simulink model "E55_1030"  (R2019b)
settings: Solver=FixedStepDiscrete  StartTime=0.0  StopTime=10  FixedStep=0.0005  RelTol=1e-3  EnableMultiTasking=on
InitFcn:
  | ecucoder_canfd
  | load('DATA_Plimit.mat')
  | a=0.775;
  | b=0.775;
  | kf=-50000;
  | kr=-50000;
  | m=226+75;
  | Iz=100;
  | u=0.85;
  | g=9.8;
  | L=a+b;
  | xi=0.1;
  | r=0.226;
  | Lw=1.171;
  | Tm=21;
  | i=15.9;
  | Jw=0.504;
  | Pmax=20000;
  | mw=19.3;
  | mb=148.9+75;
  | hg=0.280;
model workspace (MAT data in the model file):
  Initial_Steer_Position = 0
values from neighbouring files (symbols this model uses):
  SOC = [2.5 5 7.5 10 20 30 40 50 60 70 80 90 ... (14 elements, 14x1)]    [DATA_Plimit.mat]
  SOC_Discharge = [2.04592350211 2.57821618825 3.10671863859 3.63118835861 4.15200192786 4.66837694959 5.18149950051 5.69046162564 6.19532286188 6.696400261 7.19347596839 7.68712157998 ... (473 elements, 1x473)]    [DATA_Plimit.mat]
  VOLTAGE = [459.1488 476.0844 485.9448 487.344 492.822 498.8016 503.382 509.1108 518.8128 531.2472 544.5132 558.4656 ... (14 elements, 14x1)]    [DATA_Plimit.mat]
undefined symbols (not defined in the file or in its folder): DiscIntNeverNeededParam, H, HALL10, HALL6, HALL7, HALL8, HALL9, HPWM1, HPWM3, I_AN05_5V, I_AN07_5V, I_AN08_5V, I_AN09_5V, I_AN10_5V, I_SW11_H, I_SW12_H, I_SW13_H, I_SW14_H, I_SW15_H, I_SW16_H, I_SW17_H, I_SW18_H, I_SW19_H, LS1A2, O_HS1A2, O_HS1A8
libraries: ec311lib x152, simulink x92, canmsglib x30, canfdmsglib x2
(part 2 of 6)

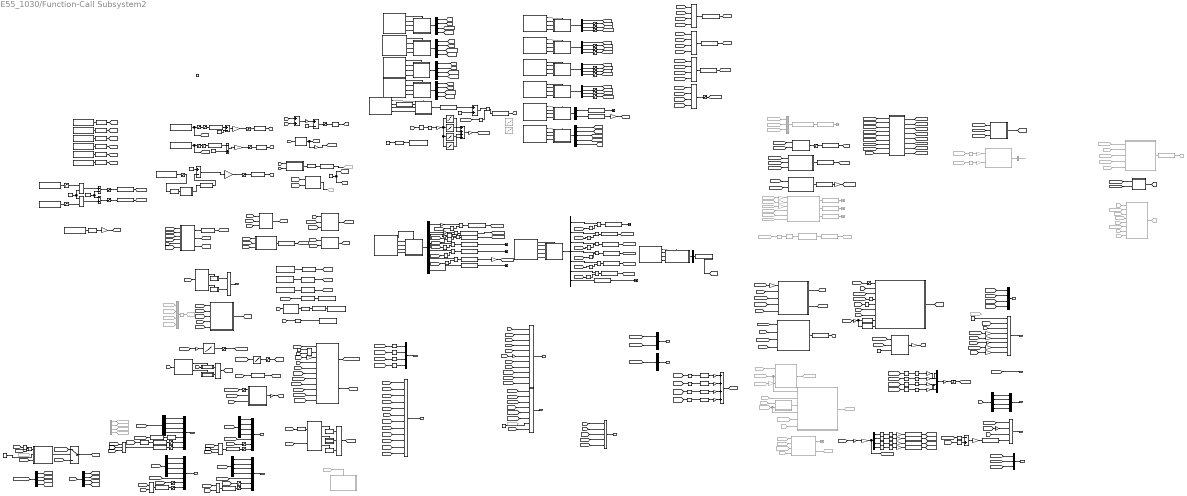
== system E55_1030/Function-Call Subsystem2 ==
  note: 三个地方要改
  note: 坐标变换（计算不带重力加速度的加速度）
  note: K3105G数据前置处理
  note: 数据滤波
  note: 此算法中量的单位：速度（m/s）、角度角速度（rad、rad/s）、轮速（rpm）
  note: 扭矩分配和驱动防滑
  note: 状态机
  note: 传感器数据接收
  note: 低压电池电压检测
  note: Yaw_Rate、Side_Slip_Angle、Steer_Angle都以向左转为正（逆时针）
  note: 设置速度
      | 待驶：0 前进：20000 倒车：-5000
  note: BMS CAN发送
  note: 功率限制
  note: 信息传输给仪表盘
  note: 精度不如IMU测的角速度
  note: 刹车油压传感器
  note: 安全回路状态检测
  note: IO输入输出
  note: 几个角度的定义，Heading和Yaw以顺时针为正，Side Slip以逆时针为正
      | Yaw Angle和Heading Angle取值为0到360°，Side Slip Angle取值为-180到180°
  note: 油门输入及可靠检测
  note: 新版CAN发送
      | 参数传入AMK
  note: 开环扭矩分配和动能回收
  note: 屏幕控制信息_55E
      | (控制K3105是否打开)
  note: 发1关闭K3105
  note: CAN接收
  note: 旋转顺序： yaw-pitch-roll
  note: XYZ：右前上
      | Yaw绕Z（左手系），Roll绕Y（右手系），Pitch绕X（右手系）
      | 加速度：XYZ正方向为负
      | Yaw：Y轴正方向和正北方向的夹角
      | Yaw_Rate：车头向左为正（右手系）
  function : TriggerPort  TriggerType=function-call  VariantControl=Variant
  1-D Lookup Table : Lookup_n-D  Commented=on  NumberOfTableDimensions=1  BreakpointsForDimension1=[-100,-60,-30.4,0,30,60,95]  Table=[-14.489,-10.473,-5.315,0,6.137,12.407,14.976]  InternalRulePriority=Speed  RndMeth=Simplest  InputSameDT=on
  1-D Lookup Table1 : Lookup_n-D  NumberOfTableDimensions=1  BreakpointsForDimension1=[0,100]  Table=[25000,36000]  InternalRulePriority=Speed  RndMeth=Simplest  InputSameDT=on
  1-D Lookup Table2 : Lookup_n-D  Commented=on  NumberOfTableDimensions=1  BreakpointsForDimension1=[-98.8,-60,-30,0,30,60,91.7]  Table=[-15.376,-12.134,-8.11,0,4.475,10.343,13.631]  InternalRulePriority=Speed  RndMeth=Simplest  InputSameDT=on
  AMKSpeed10 : canmsglib/CAN Pack  Commented=on  MsgList=(none)  MsgName=ESC_5_RearWhlSpdKPH  MsgIDType=Standard (11-bit identifier)  MsgIdentifier=291  MsgLength=8  Remote=off  ApplyMinMax=off  BusOutput=on  SignalInfo={ 'ESC_WheelSpeedKph_RL', '8', '13', 'BE', 'unsigned', 'Standard', '0', '0.05625', '0', '0', '460.6875'; 'ESC_WheelSpeedKph_RR', '24', '13', 'BE', 'unsigned', 'Standard', '0', '0.05625', '0', '0', '460.6875' }
      settings: SourceProductName=Vehicle Network Toolbox  SourceProductBaseCode=VN  DataFormat=manually specified signals
  AMK复位开关 : ec311lib/RapidECU_U34/01BasicInput/SwitchInput  channel=103:I_SW19_H/HALL10  sampletime=-1
      settings: SourceProductName=ECUCoder for S32K311
  Abs{,1..7} (8 alike) : Abs
  Abs10 : Abs  Commented=on
  Abs8 : Abs  Commented=on
  Abs9 : Abs  Commented=on
  Add : Sum  Inputs=++++
  Add1 : Sum
  Add2 : Sum  Inputs=+-
  Add3 : Sum  Inputs=+-
  Add4 : Sum  Inputs=-+
  Add5 : Sum
  AnalogInput : ec311lib/RapidECU_U34/01BasicInput/AnalogInput  channel=55:I_AN08_5V  sampletime=-1
      settings: SourceProductName=ECUCoder for S32K311
  AnalogInput1 : ec311lib/RapidECU_U34/01BasicInput/AnalogInput  channel=56:I_AN09_5V  sampletime=-1
      settings: SourceProductName=ECUCoder for S32K311
  BRAKE_HIGH1 : Constant  Value=1153
  Bus Creator{,6..7,14} (4 alike) : BusCreator  Inputs=4
  Bus Creator{1..4} (4 alike) : BusCreator  Inputs=7
  Bus Creator10 : BusCreator  Inputs=8
  Bus Creator11 : BusCreator  Inputs=1
  Bus Creator12 : BusCreator  Inputs=2
  Bus Creator13 : BusCreator  Inputs=3
  Bus Creator15 : BusCreator  Inputs=5
  Bus Creator5 : BusCreator  Inputs=8
  Bus Creator8 : BusCreator  Inputs=12
  Bus Creator9 : BusCreator  Inputs=11
  Bus Selector : BusSelector  OutputSignals=K3105_Alive
  Bus Selector1 : BusSelector  OutputSignals=INS_IMUAccrnX,INS_IMUAccrnY,INS_IMUAccrnZ,INS_IMUAglRateX,INS_IMUAglRateY,INS_IMUAglRateZ,CAN_OK
  Bus Selector{8..11} (4 alike) : BusSelector  OutputSignals=ErrorCode,TempIGBT,TempInverter,TempMotor
  Bus Selector12 : BusSelector  OutputSignals=IVT_MsgCount,IVT_Msg_Result_W
  Bus Selector13 : BusSelector  OutputSignals=BMSState,CellTemp,MaxCellVolt,MinCellVolt,SOC
  Bus Selector{18,20,22,24} (4 alike) : BusSelector  OutputSignals=DcOn,Enable,ErrorReset,InverterOn
  Bus Selector2 : BusSelector  OutputSignals=To_Ground_Speed,East_Speed,North_Speed,Heading_Angle,Pitch_Angle,Roll_Angle,CAN_OK
  Bus Selector27 : BusSelector  Commented=on  OutputSignals=Data
  Bus Selector{3..6} (4 alike) : BusSelector  OutputSignals=Id,Iq,AMK_Speed,bError
  CAN0to2Receive : ec311lib/RapidECU_U34/03CANCommunication/CAN0to2Receive  canmodule=2  canbuffer=56  canmessageid=hex2dec('0283')  canmessagetype=Standard(11-bit ID)  datalength=8  sampletime=-1
      settings: SourceProductName=ECUCoder for S32K311
  CAN0to2Receive1 : ec311lib/RapidECU_U34/03CANCommunication/CAN0to2Receive  canmodule=2  canbuffer=57  canmessageid=hex2dec('0284')  canmessagetype=Standard(11-bit ID)  datalength=8  sampletime=-1
      settings: SourceProductName=ECUCoder for S32K311
  CAN0to2Receive10 : ec311lib/RapidECU_U34/03CANCommunication/CAN0to2Receive  canmodule=0  canbuffer=20  canmessageid=hex2dec('055A')  canmessagetype=Standard(11-bit ID)  datalength=8  sampletime=-1
      settings: SourceProductName=ECUCoder for S32K311
  CAN0to2Receive13 : ec311lib/RapidECU_U34/03CANCommunication/CAN0to2Receive  canmodule=0  canbuffer=21  canmessageid=hex2dec('055E')  canmessagetype=Standard(11-bit ID)  datalength=8  sampletime=-1
      settings: SourceProductName=ECUCoder for S32K311
  CAN0to2Receive2 : ec311lib/RapidECU_U34/03CANCommunication/CAN0to2Receive  canmodule=2  canbuffer=58  canmessageid=hex2dec('0287')  canmessagetype=Standard(11-bit ID)  datalength=8  sampletime=-1
      settings: SourceProductName=ECUCoder for S32K311
  CAN0to2Receive3 : ec311lib/RapidECU_U34/03CANCommunication/CAN0to2Receive  canmodule=2  canbuffer=59  canmessageid=hex2dec('0288')  canmessagetype=Standard(11-bit ID)  datalength=8  sampletime=-1
      settings: SourceProductName=ECUCoder for S32K311
  CAN0to2Receive4 : ec311lib/RapidECU_U34/03CANCommunication/CAN0to2Receive  canmodule=2  canbuffer=60  canmessageid=hex2dec('0285')  canmessagetype=Standard(11-bit ID)  datalength=8  sampletime=-1
      settings: SourceProductName=ECUCoder for S32K311
  CAN0to2Receive5 : ec311lib/RapidECU_U34/03CANCommunication/CAN0to2Receive  canmodule=2  canbuffer=61  canmessageid=hex2dec('0286')  canmessagetype=Standard(11-bit ID)  datalength=8  sampletime=-1
      settings: SourceProductName=ECUCoder for S32K311
  CAN0to2Receive6 : ec311lib/RapidECU_U34/03CANCommunication/CAN0to2Receive  canmodule=2  canbuffer=62  canmessageid=hex2dec('0289')  canmessagetype=Standard(11-bit ID)  datalength=8  sampletime=-1
      settings: SourceProductName=ECUCoder for S32K311
  CAN0to2Receive7 : ec311lib/RapidECU_U34/03CANCommunication/CAN0to2Receive  canmodule=2  canbuffer=63  canmessageid=hex2dec('028A')  canmessagetype=Standard(11-bit ID)  datalength=8  sampletime=-1
      settings: SourceProductName=ECUCoder for S32K311
  CAN0to2Receive8 : ec311lib/RapidECU_U34/03CANCommunication/CAN0to2Receive  canmodule=0  canbuffer=35  canmessageid=hex2dec('01E5')  canmessagetype=Standard(11-bit ID)  datalength=8  sampletime=-1
      settings: SourceProductName=ECUCoder for S32K311
  CAN0to2Receive9 : ec311lib/RapidECU_U34/03CANCommunication/CAN0to2Receive  canmodule=0  canbuffer=24  canmessageid=hex2dec('0526')  canmessagetype=Standard(11-bit ID)  datalength=6  sampletime=-1
      settings: SourceProductName=ECUCoder for S32K311
  CAN5WakeUp : ec311lib/RapidECU_U34/03CANCommunication/CAN5WakeUp  channel=CAN5WakeUp  sampletime=-1
      settings: SourceProductName=ECUCoder for S32K311
  Constant{,5..7} (4 alike) : Constant
  Constant10 : Constant  Value=0
  Constant11 : Constant  Value=0
  Constant2 : Constant  Value=-377
  Constant25 : Constant  Value=3.125
  Constant3 : Constant  Value=3271
  Constant36 : Constant  Value=160
  Constant4 : Constant  Value=5
  Constant8 : Constant  Value=0
  Constant9 : Constant  Value=1433
  Data Type Conversion{,1,5,7..9,12..13} (8 alike) : DataTypeConversion
  Data Type Conversion10 : DataTypeConversion  OutDataTypeStr=boolean
  Data Type Conversion11 : DataTypeConversion  OutDataTypeStr=int16  RndMeth=Nearest
  Data Type Conversion14 : DataTypeConversion  OutDataTypeStr=boolean
  Data Type Conversion2 : DataTypeConversion  RndMeth=Nearest
  Data Type Conversion6 : DataTypeConversion  OutDataTypeStr=boolean
  Demux{,1,3..4} (4 alike) : Demux
  Demux2 : Demux  Commented=on
  Difference : simulink/Discrete/Difference  Commented=on  ICPrevInput=0.0  OutMin=[]  OutMax=[]  OutDataType=fixdt(1, 16)  OutScaling=2^-10  DoSatur=off
  Divide5 : Product  Inputs=/*
  Divide7 : Product  Inputs=*/
  Fcn1 : Fcn  Commented=on  Expr=sqrt(u(1)*u(1)+u(2)*u(2)+u(3)*u(3))
  From15 : From  Commented=on  GotoTag=reset_input
  From158 : From  Commented=on  GotoTag=Wheel_Steer_Angle
  From170 : From  Commented=on  GotoTag=Yaw_Rate_d
  From171 : From  Commented=on  GotoTag=wheel_speed_d
  From172 : From  Commented=on  GotoTag=wheel_speed_d
  From174 : From  Commented=on  GotoTag=wheel_speed
  From177 : From  Commented=on  GotoTag=velocity
  From182 : From  Commented=on  GotoTag=wheel_speed
  From183 : From  Commented=on  GotoTag=Torque_Dis
  From184 : From  Commented=on  GotoTag=Torque_ASR
  From197 : From  Commented=on  GotoTag=T_max_d
  From207 : From  Commented=on  GotoTag=INS_IMUAccrnY_filter
  From221 : From  Commented=on  GotoTag=Algorithm_Enable
  From224 : From  Commented=on  GotoTag=Algorithm_Enable
  From232 : From  Commented=on  GotoTag=AMKSpeed_RR
  From233 : From  Commented=on  GotoTag=AMKSpeed_FL
  From234 : From  Commented=on  GotoTag=AMKSpeed_FR
  From235 : From  Commented=on  GotoTag=AMKSpeed_RL
  From239 : From  Commented=on  GotoTag=Yaw_Rate_d
  From240 : From  Commented=on  GotoTag=Yaw_Rate_d
  From241 : From  Commented=on  GotoTag=Wheel_Steer_Angle
  From242 : From  Commented=on  GotoTag=velocity
  From243 : From  Commented=on  GotoTag=Side_Slip_Angle
  From244 : From  Commented=on  GotoTag=Yaw_Rate_filter
  From245 : From  Commented=on  GotoTag=Fz
  From246 : From  Commented=on  GotoTag=break
  From247 : From  Commented=on  GotoTag=Wheel_Steer_Angle
  From248 : From  Commented=on  GotoTag=Torque_req
  From25 : From  Commented=on  GotoTag=INS_IMUAccrnX
  From252 : From  Commented=on  GotoTag=T_max_d
  From255 : From  Commented=on  GotoTag=Mz_r
  From26 : From  Commented=on  GotoTag=Yaw_Rate_filter
  From27 : From  Commented=on  GotoTag=INS_IMUAccrnY
  From28 : From  Commented=on  GotoTag=INS_IMUAccrnZ
  From29 : From  Commented=on  GotoTag=Yaw_Angle
  From33 : From  Commented=on  GotoTag=AMKSpeed_RR
  From34 : From  Commented=on  GotoTag=Torque_Dis
  From37 : From  Commented=on  GotoTag=Pitch_Angle_filter
  From38 : From  Commented=on  GotoTag=Roll_Angle_filter
  From39 : From  Commented=on  GotoTag=INS_IMUAccrnX_filter
  From41 : From  Commented=on  GotoTag=Yaw_Rate_filter
  From42 : From  Commented=on  GotoTag=INS_IMUAccrnZ
  From47 : From  Commented=on  GotoTag=Yaw_Angle_filter
  From90 : From  Commented=on  GotoTag=AMKSpeed_RL
  From94 : From  Commented=on  GotoTag=Algorithm_Enable
  Function-Call Subsystem : Subsystem  TreatAsAtomicUnit=on
  Gain{10,49..51} (4 alike) : Gain
  Gain11 : Gain  Commented=on  Gain=(2*pi*r*3.6)/(60*i)
  Gain{14..16,35} (4 alike) : Gain  Commented=on  Gain=pi/180
  Gain17 : Gain  Gain=3.6
  Gain18 : Gain  Gain=1/9.8
  Gain19 : Gain  Gain=0.01
  Gain2 : Gain  Gain=0.001  OutDataTypeStr=Inherit: Inherit via back propagation
  Gain21 : Gain  Gain=0.95
  Gain22 : Gain  Gain=pi/180
  Gain23 : Gain  Gain=0.5
  Gain25 : Gain  Gain=1/i
  Gain{26..29} (4 alike) : Gain  Gain=1/2
  Gain3 : Gain  Commented=on  Gain=(2*pi*r*3.6)/(60*i)
  Gain30 : Gain  Gain=100
  Gain31 : Gain  Gain=1/10
  Gain32 : Gain  Gain=1/4
  Gain{33,39..41} (4 alike) : Gain  Gain=1/40
  Gain34 : Gain  Gain=1/i
  Gain36 : Gain  Gain=pi/180
  Gain37 : Gain  Gain=0.95
  Gain38 : Gain  Gain=1000/9.8
  Gain4 : Gain  Gain=132
  Gain{42..44,46..47} (5 alike) : Gain  Gain=180/pi
  Gain45 : Gain  Gain=3.6
  Gain48 : Gain  Gain=100
  Gain52 : Gain  Gain=pi/180
  Gain6 : Gain  Gain=0.001
  Gain7 : Gain  Gain=8
  Gain8 : Gain  Gain=4
  Gain9 : Gain  Gain=2
  Goto : Goto  Commented=on  GotoTag=AMKSpeed
  Goto118 : Goto  Commented=on  GotoTag=ASR_Status
  Goto120 : Goto  Commented=on  GotoTag=TargetVelocity_FR
  Goto121 : Goto  Commented=on  GotoTag=TargetVelocity_RL
  Goto122 : Goto  Commented=on  GotoTag=TargetVelocity_RR
  Goto124 : Goto  Commented=on  GotoTag=Mz_r
  Goto125 : Goto  Commented=on  GotoTag=Tx
  Goto137 : Goto  Commented=on  GotoTag=acc_flag
  Goto138 : Goto  Commented=on  GotoTag=acc_out
  Goto23 : Goto  Commented=on  GotoTag=TargetVelocity_FL
  Goto29 : Goto  Commented=on  GotoTag=Yaw_Rate
  Goto45 : Goto  Commented=on  GotoTag=wheel_speed_d
  Goto46 : Goto  Commented=on  GotoTag=Torque_ASR
  If Action Subsystem15 : Subsystem  TreatAsAtomicUnit=on
  If Action Subsystem16 : Subsystem  TreatAsAtomicUnit=on
  If Action Subsystem20 : Subsystem  TreatAsAtomicUnit=on
  If Action Subsystem21 : Subsystem  TreatAsAtomicUnit=on
  If Action Subsystem22 : Subsystem  TreatAsAtomicUnit=on
  If Action Subsystem5 : Subsystem  TreatAsAtomicUnit=on
  If Action Subsystem7 : Subsystem  TreatAsAtomicUnit=on
  If Action Subsystem9 : Subsystem  TreatAsAtomicUnit=on
  If3 : If  IfExpression=u1 > 1
  If7 : If  IfExpression=u1<6.66
  If9 : If  NumInputs=2  ElseIfExpressions=u2 == 3
  Logical Operator{1..13,15} (14 alike) : Logic  Operator=NOT  AllPortsSameDT=off  OutDataTypeStr=boolean
  Logical Operator14 : Logic  AllPortsSameDT=off  OutDataTypeStr=boolean
  M64CAN3to5Receive2 : ec311lib/RapidECU_U34/04CANFDCommunication/Max64Bytes/M64CAN3to5Receive  canmodule=5  canbuffer=0  canmessageid=hex2dec('00FC')  canmessagetype=Standard(11-bit ID)  datalength=64  unpack=on  sampletime=-1
      settings: SourceProductName=ECUCoder for S32K311
  M64CAN3to5Receive3 : ec311lib/RapidECU_U34/04CANFDCommunication/Max64Bytes/M64CAN3to5Receive  canmodule=5  canbuffer=1  canmessageid=hex2dec('00FD')  canmessagetype=Standard(11-bit ID)  datalength=64  unpack=on  sampletime=-1
      settings: SourceProductName=ECUCoder for S32K311
  MATLAB Function : MATLAB Function  TreatAsAtomicUnit=on
  MATLAB Function1 : MATLAB Function  TreatAsAtomicUnit=on
  MATLAB Function10 : MATLAB Function  TreatAsAtomicUnit=on
  MATLAB Function11 : MATLAB Function  TreatAsAtomicUnit=on
  MATLAB Function12 : MATLAB Function  TreatAsAtomicUnit=on
  MATLAB Function13 : MATLAB Function  TreatAsAtomicUnit=on
  MATLAB Function14 : MATLAB Function  TreatAsAtomicUnit=on
  MATLAB Function16 : MATLAB Function  TreatAsAtomicUnit=on
  MATLAB Function2 : MATLAB Function  Commented=on  TreatAsAtomicUnit=on
  MATLAB Function3 : MATLAB Function  Commented=on  TreatAsAtomicUnit=on
  MATLAB Function4 : MATLAB Function  TreatAsAtomicUnit=on
  MATLAB Function5 : MATLAB Function  TreatAsAtomicUnit=on
  MATLAB Function6 : MATLAB Function  TreatAsAtomicUnit=on
  MATLAB Function7 : MATLAB Function  TreatAsAtomicUnit=on
  MATLAB Function8 : MATLAB Function  TreatAsAtomicUnit=on
  MATLAB Function9 : MATLAB Function  TreatAsAtomicUnit=on
  Max{,1..3} (4 alike) : MinMax  Function=max  Inputs=4
  MeaModule : ec311lib/RapidECU_U34/09Calibration/MeaModule  signal=acc
      settings: SourceProductName=ECUCoder for S32K311
  MeaModule1 : ec311lib/RapidECU_U34/09Calibration/MeaModule  signal=acc2_input
      settings: SourceProductName=ECUCoder for S32K311
  MeaModule10 : ec311lib/RapidECU_U34/09Calibration/MeaModule  signal=Steer
      settings: SourceProductName=ECUCoder for S32K311
  MeaModule11 : ec311lib/RapidECU_U34/09Calibration/MeaModule  signal=acc2
      settings: SourceProductName=ECUCoder for S32K311
  MeaModule12 : ec311lib/RapidECU_U34/09Calibration/MeaModule  signal=acc1
      settings: SourceProductName=ECUCoder for S32K311
  MeaModule13 : ec311lib/RapidECU_U34/09Calibration/MeaModule  signal=brake_output
      settings: SourceProductName=ECUCoder for S32K311
  MeaModule14 : ec311lib/RapidECU_U34/09Calibration/MeaModule  signal=Algorithm_Enable
      settings: SourceProductName=ECUCoder for S32K311
  MeaModule15 : ec311lib/RapidECU_U34/09Calibration/MeaModule  signal=Steer_CANOK
      settings: SourceProductName=ECUCoder for S32K311
  MeaModule16 : ec311lib/RapidECU_U34/09Calibration/MeaModule  signal=delta_YawRate
      settings: SourceProductName=ECUCoder for S32K311
  MeaModule17 : ec311lib/RapidECU_U34/09Calibration/MeaModule  signal=DeratingRatio
      settings: SourceProductName=ECUCoder for S32K311
  MeaModule19 : ec311lib/RapidECU_U34/09Calibration/MeaModule  signal=BreakPressure_F
      settings: SourceProductName=ECUCoder for S32K311
  MeaModule2 : ec311lib/RapidECU_U34/09Calibration/MeaModule  signal=run_flag
      settings: SourceProductName=ECUCoder for S32K311
  MeaModule20 : ec311lib/RapidECU_U34/09Calibration/MeaModule  signal=break_transmit
      settings: SourceProductName=ECUCoder for S32K311
  MeaModule21 : ec311lib/RapidECU_U34/09Calibration/MeaModule  signal=Power
      settings: SourceProductName=ECUCoder for S32K311
  MeaModule22 : ec311lib/RapidECU_U34/09Calibration/MeaModule  signal=IVT_MsgCount
      settings: SourceProductName=ECUCoder for S32K311
  MeaModule23 : ec311lib/RapidECU_U34/09Calibration/MeaModule  signal=Torque_FR_out
      settings: SourceProductName=ECUCoder for S32K311
  MeaModule25 : ec311lib/RapidECU_U34/09Calibration/MeaModule  Commented=on  signal=Mz_r
      settings: SourceProductName=ECUCoder for S32K311
  MeaModule26 : ec311lib/RapidECU_U34/09Calibration/MeaModule  signal=reset_input
      settings: SourceProductName=ECUCoder for S32K311
  MeaModule27 : ec311lib/RapidECU_U34/09Calibration/MeaModule  signal=BreakPressure_R
      settings: SourceProductName=ECUCoder for S32K311
  MeaModule29 : ec311lib/RapidECU_U34/09Calibration/MeaModule  signal=readyLED_output
      settings: SourceProductName=ECUCoder for S32K311
  MeaModule31 : ec311lib/RapidECU_U34/09Calibration/MeaModule  signal=TargetVelocity
      settings: SourceProductName=ECUCoder for S32K311
  MeaModule32 : ec311lib/RapidECU_U34/09Calibration/MeaModule  signal=NegTorque
      settings: SourceProductName=ECUCoder for S32K311
  MeaModule33 : ec311lib/RapidECU_U34/09Calibration/MeaModule  signal=Torque_RR_out
      settings: SourceProductName=ECUCoder for S32K311
  MeaModule4 : ec311lib/RapidECU_U34/09Calibration/MeaModule  signal=brake_input
      settings: SourceProductName=ECUCoder for S32K311
  MeaModule40 : ec311lib/RapidECU_U34/09Calibration/MeaModule  Commented=on  signal=acc_including_g
      settings: SourceProductName=ECUCoder for S32K311
  MeaModule41 : ec311lib/RapidECU_U34/09Calibration/MeaModule  Commented=on  signal=Yaw_Rate
      settings: SourceProductName=ECUCoder for S32K311
  MeaModule42 : ec311lib/RapidECU_U34/09Calibration/MeaModule  signal=Heading_Angle
      settings: SourceProductName=ECUCoder for S32K311
  MeaModule43 : ec311lib/RapidECU_U34/09Calibration/MeaModule  Commented=on  signal=Acc_X
      settings: SourceProductName=ECUCoder for S32K311
  MeaModule44 : ec311lib/RapidECU_U34/09Calibration/MeaModule  Commented=on  signal=Acc_Y
      settings: SourceProductName=ECUCoder for S32K311
  MeaModule45 : ec311lib/RapidECU_U34/09Calibration/MeaModule  Commented=on  signal=Acc_Z
      settings: SourceProductName=ECUCoder for S32K311
  MeaModule46 : ec311lib/RapidECU_U34/09Calibration/MeaModule  signal=SC_State
      settings: SourceProductName=ECUCoder for S32K311
  MeaModule47 : ec311lib/RapidECU_U34/09Calibration/MeaModule  signal=SC_Testpoint1
      settings: SourceProductName=ECUCoder for S32K311
  MeaModule48 : ec311lib/RapidECU_U34/09Calibration/MeaModule  signal=SC_Testpoint2
      settings: SourceProductName=ECUCoder for S32K311
  MeaModule49 : ec311lib/RapidECU_U34/09Calibration/MeaModule  signal=SC_Testpoint3
      settings: SourceProductName=ECUCoder for S32K311
  MeaModule5 : ec311lib/RapidECU_U34/09Calibration/MeaModule  signal=start_input
      settings: SourceProductName=ECUCoder for S32K311
  MeaModule50 : ec311lib/RapidECU_U34/09Calibration/MeaModule  signal=SC_Testpoint4
      settings: SourceProductName=ECUCoder for S32K311
  MeaModule51 : ec311lib/RapidECU_U34/09Calibration/MeaModule  signal=SC_Testpoint5
      settings: SourceProductName=ECUCoder for S32K311
  MeaModule52 : ec311lib/RapidECU_U34/09Calibration/MeaModule  signal=MaxTempInverter_n
      settings: SourceProductName=ECUCoder for S32K311
  MeaModule53 : ec311lib/RapidECU_U34/09Calibration/MeaModule  signal=MaxTempMotor_n
      settings: SourceProductName=ECUCoder for S32K311
  MeaModule54 : ec311lib/RapidECU_U34/09Calibration/MeaModule  signal=Side_Slip_Angle
      settings: SourceProductName=ECUCoder for S32K311
  MeaModule55 : ec311lib/RapidECU_U34/09Calibration/MeaModule  signal=velocity
      settings: SourceProductName=ECUCoder for S32K311
  MeaModule6 : ec311lib/RapidECU_U34/09Calibration/MeaModule  signal=MaxTempIGBT_n
      settings: SourceProductName=ECUCoder for S32K311
  MeaModule61 : ec311lib/RapidECU_U34/09Calibration/MeaModule  signal=INS_IMUAccrnZ
      settings: SourceProductName=ECUCoder for S32K311
  MeaModule62 : ec311lib/RapidECU_U34/09Calibration/MeaModule  signal=Torque_FR
      settings: SourceProductName=ECUCoder for S32K311
  MeaModule63 : ec311lib/RapidECU_U34/09Calibration/MeaModule  signal=Torque_FL
      settings: SourceProductName=ECUCoder for S32K311
  MeaModule64 : ec311lib/RapidECU_U34/09Calibration/MeaModule  signal=Torque_RR
      settings: SourceProductName=ECUCoder for S32K311
  MeaModule65 : ec311lib/RapidECU_U34/09Calibration/MeaModule  signal=Torque_RL
      settings: SourceProductName=ECUCoder for S32K311
  MeaModule66 : ec311lib/RapidECU_U34/09Calibration/MeaModule  signal=Raw_Steer
      settings: SourceProductName=ECUCoder for S32K311
  MeaModule67 : ec311lib/RapidECU_U34/09Calibration/MeaModule  signal=INS_IMUAglRateX
      settings: SourceProductName=ECUCoder for S32K311
  MeaModule68 : ec311lib/RapidECU_U34/09Calibration/MeaModule  signal=Mz
      settings: SourceProductName=ECUCoder for S32K311
  MeaModule69 : ec311lib/RapidECU_U34/09Calibration/MeaModule  signal=Torque_FL_out
      settings: SourceProductName=ECUCoder for S32K311
  MeaModule7 : ec311lib/RapidECU_U34/09Calibration/MeaModule  signal=acc1_input
      settings: SourceProductName=ECUCoder for S32K311
  MeaModule70 : ec311lib/RapidECU_U34/09Calibration/MeaModule  signal=Torque_RL_out
      settings: SourceProductName=ECUCoder for S32K311
  MeaModule71 : ec311lib/RapidECU_U34/09Calibration/MeaModule  signal=INS_IMUAglRateY
      settings: SourceProductName=ECUCoder for S32K311
  MeaModule72 : ec311lib/RapidECU_U34/09Calibration/MeaModule  signal=Yaw_Rate
      settings: SourceProductName=ECUCoder for S32K311
  MeaModule73 : ec311lib/RapidECU_U34/09Calibration/MeaModule  signal=CAN_OK_IMU
      settings: SourceProductName=ECUCoder for S32K311
  MeaModule74 : ec311lib/RapidECU_U34/09Calibration/MeaModule  signal=INS_IMUAccrnX
      settings: SourceProductName=ECUCoder for S32K311
  MeaModule75 : ec311lib/RapidECU_U34/09Calibration/MeaModule  signal=To_Ground_Speed
      settings: SourceProductName=ECUCoder for S32K311
  MeaModule76 : ec311lib/RapidECU_U34/09Calibration/MeaModule  signal=CAN_OK_GNSS
      settings: SourceProductName=ECUCoder for S32K311
  MeaModule77 : ec311lib/RapidECU_U34/09Calibration/MeaModule  signal=Yaw_Angle
      settings: SourceProductName=ECUCoder for S32K311
  MeaModule78 : ec311lib/RapidECU_U34/09Calibration/MeaModule  signal=East_Speed
      settings: SourceProductName=ECUCoder for S32K311
  MeaModule79 : ec311lib/RapidECU_U34/09Calibration/MeaModule  signal=North_Speed
      settings: SourceProductName=ECUCoder for S32K311
  MeaModule8 : ec311lib/RapidECU_U34/09Calibration/MeaModule  signal=precharge_input
      settings: SourceProductName=ECUCoder for S32K311
  MeaModule80 : ec311lib/RapidECU_U34/09Calibration/MeaModule  signal=Pitch_Angle
      settings: SourceProductName=ECUCoder for S32K311
  MeaModule81 : ec311lib/RapidECU_U34/09Calibration/MeaModule  signal=Roll_Angle
      settings: SourceProductName=ECUCoder for S32K311
  MeaModule82 : ec311lib/RapidECU_U34/09Calibration/MeaModule  signal=INS_IMUAccrnY
      settings: SourceProductName=ECUCoder for S32K311
  MeaModule83 : ec311lib/RapidECU_U34/09Calibration/MeaModule  signal=K3105_Alive
      settings: SourceProductName=ECUCoder for S32K311
  MeaModule9 : ec311lib/RapidECU_U34/09Calibration/MeaModule  signal=acc_flag
      settings: SourceProductName=ECUCoder for S32K311
  Merge4 : Merge
  Merge6 : Merge  Inputs=3
  Merge8 : Merge
  Mux1 : Mux  Commented=on  Inputs=3
  Mux2 : Mux  Commented=on
  Mux3 : Mux
  NOT{,1..3} (4 alike) : Logic  Operator=NOT  IconShape=distinctive  AllPortsSameDT=off  OutDataTypeStr=boolean
  PowerDriverSwitch(HS) : ec311lib/RapidECU_U34/02BasicOutput/PowerDriverSwitch(HS)  channel=117:O_HS1A8/HPWM3  sampletime=-1
      settings: SourceProductName=ECUCoder for S32K311
  PowerDriverSwitch(HS)1 : ec311lib/RapidECU_U34/02BasicOutput/PowerDriverSwitch(HS)  channel=115:O_HS1A2/HPWM2/LS1A2  sampletime=-1
      settings: SourceProductName=ECUCoder for S32K311
  PowerDriverSwitch(HS)2 : ec311lib/RapidECU_U34/02BasicOutput/PowerDriverSwitch(HS)  channel=114:O_HS1A2/HPWM1/LS1A2/H+  sampletime=-1
      settings: SourceProductName=ECUCoder for S32K311
  PowerVoltageMonitor : ec311lib/RapidECU_U34/07PowerManagement/PowerVoltageMonitor  channel=4-5: I_BAT  sampletime=-1
      settings: SourceProductName=ECUCoder for S32K311
  Product : Product  Inputs=3
  Product{1,3..17} (16 alike) : Product
  Product2 : Product  Inputs=3
  SMC : Subsystem
  SMC_ASR : Subsystem  Commented=on
  SMC_yaw_rate : Subsystem  Commented=on
  Saturation{,1..2,5} (4 alike) : Saturate  UpperLimit=2140  LowerLimit=0
  Saturation{3..4,9..10} (4 alike) : Saturate  UpperLimit=5000  LowerLimit=0  OutDataTypeStr=double
  Saturation{11..22} (12 alike) : Saturate  UpperLimit=1200  LowerLimit=0
  Saturation{6,23..25} (4 alike) : Saturate  UpperLimit=0  LowerLimit=-1000
  Saturation26 : Saturate  UpperLimit=100  LowerLimit=0
  Saturation27 : Saturate  UpperLimit=25  LowerLimit=0  OutDataTypeStr=double
  Saturation28 : Saturate  UpperLimit=25  LowerLimit=0  OutDataTypeStr=double
  Saturation29 : Saturate  UpperLimit=20000  LowerLimit=0.1
  Saturation30 : Saturate  UpperLimit=1300  LowerLimit=0.1
  Saturation31 : Saturate  UpperLimit=200  LowerLimit=0
  Saturation32 : Saturate  UpperLimit=105  LowerLimit=0
  Saturation33 : Saturate  UpperLimit=105  LowerLimit=0
  Saturation34 : Saturate  UpperLimit=100  LowerLimit=0
  Saturation35 : Saturate  UpperLimit=100  LowerLimit=0
  Saturation36 : Saturate  UpperLimit=3900  LowerLimit=3271
  Saturation37 : Saturate  UpperLimit=1433  LowerLimit=768
  Saturation38 : Saturate  UpperLimit=33  LowerLimit=0
  Saturation39 : Saturate  UpperLimit=1  LowerLimit=0
  Saturation40 : Saturate  UpperLimit=20000  LowerLimit=0
  Saturation41 : Saturate  UpperLimit=5000  LowerLimit=0
  StateChange1 : Stateflow chart  TreatAsAtomicUnit=on
  StateChange2 : Stateflow chart  TreatAsAtomicUnit=on
  StateChange3 : Stateflow chart  TreatAsAtomicUnit=on
  StateChange4 : Stateflow chart  TreatAsAtomicUnit=on
  StateChange5 : Stateflow chart  TreatAsAtomicUnit=on
  Subsystem : Subsystem
  Subsystem1 : Subsystem
  Subsystem10 : Subsystem
  Subsystem11 : Subsystem
  Subsystem12 : Subsystem
  Subsystem15 : Subsystem
  Subsystem17 : Subsystem  Commented=on
  Subsystem18 : Subsystem
  Subsystem19 : Subsystem
  Subsystem2 : Subsystem
  Subsystem3 : Subsystem
  Subsystem4 : Subsystem
  Subsystem5 : Subsystem
  Subsystem6 : Subsystem
  Subsystem7 : Subsystem
  Subsystem8 : Subsystem
  Subtract1 : Sum  Inputs=+-
  Subtract11 : Sum  Inputs=+-
  Subtract2 : Sum  Inputs=-+
  Subtract3 : Sum  Inputs=-+
  Subtract8 : Sum  Inputs=++++
  Sum of Elements{,1..8} (9 alike) : Sum  Inputs=+
  Switch : Switch  Criteria=u2 ~= 0  Threshold=0.05
  SwitchInput10 : ec311lib/RapidECU_U34/01BasicInput/SwitchInput  channel=100:I_SW17_H  sampletime=-1
      settings: SourceProductName=ECUCoder for S32K311
  SwitchInput11 : ec311lib/RapidECU_U34/01BasicInput/SwitchInput  channel=38:I_SW11_H/HALL6  sampletime=-1
      settings: SourceProductName=ECUCoder for S32K311
  SwitchInput6 : ec311lib/RapidECU_U34/01BasicInput/SwitchInput  channel=39:I_SW12_H/HALL7  sampletime=-1
      settings: SourceProductName=ECUCoder for S32K311
  SwitchInput7 : ec311lib/RapidECU_U34/01BasicInput/SwitchInput  channel=44:I_SW14_H  sampletime=-1
      settings: SourceProductName=ECUCoder for S32K311
  SwitchInput8 : ec311lib/RapidECU_U34/01BasicInput/SwitchInput  channel=46:I_SW15_H  sampletime=-1
      settings: SourceProductName=ECUCoder for S32K311
  SwitchInput9 : ec311lib/RapidECU_U34/01BasicInput/SwitchInput  channel=65:I_SW16_H  sampletime=-1
      settings: SourceProductName=ECUCoder for S32K311
  Tapped Delay{,1..3} (4 alike) : simulink/Discrete/Tapped Delay  vinit=0.0  samptime=-1  NumDelays=2  DelayOrder=Oldest  includeCurrent=off
  Tapped Delay4 : simulink/Discrete/Tapped Delay  vinit=0.0  samptime=-1  NumDelays=10  DelayOrder=Oldest  includeCurrent=off
  Tapped Delay{5..8} (4 alike) : simulink/Discrete/Tapped Delay  vinit=0.0  samptime=-1  NumDelays=40  DelayOrder=Oldest  includeCurrent=off
  Terminator{2,10..11,16..17} (5 alike) : Terminator  Commented=on
  Terminator{4,7..9,12..13} (6 alike) : Terminator
  Triggered Subsystem : Subsystem  Commented=on  TreatAsAtomicUnit=on
  Zero-Order Hold : ZeroOrderHold  Commented=on  SampleTime=0.1
  left1 : Lookup_n-D  NumberOfTableDimensions=1  BreakpointsForDimension1=VOLTAGE  BreakpointsForDimension2=[400;403;406;409;412;415;418;421;424;427;430;433;436;439;442;445;448;451;454;457;460;463;466;469;472;475;478;481;484;487;490;493;496;499;502;505;508;511;514;517;520;523;526;529;532;535;538;541;544;547;550;553;556;559;562;565;568;571]  Table=SOC  InternalRulePriority=Speed  RndMeth=Simplest  InputSameDT=on
  mV_to % : Gain  Gain=100/764
  mV_to %1 : Gain  Gain=105/768
  mV_to %2 : Gain  Gain=105/629
  刹车输入 : ec311lib/RapidECU_U34/01BasicInput/AnalogInput  channel=71:I_AN10_5V  sampletime=-1
      settings: SourceProductName=ECUCoder for S32K311
  功率限制 : Subsystem
  功率限制1 : Subsystem
  右轮上行 : Lookup_n-D  NumberOfTableDimensions=1  BreakpointsForDimension1=[-100,-60,-30,0,30,60,85,95]  Table=[-13.8,-10.15,-6.1,0.15,6.85,13.35,15.7,15.7]  InternalRulePriority=Speed  RndMeth=Simplest  InputSameDT=on
  右轮下行 : Lookup_n-D  NumberOfTableDimensions=1  BreakpointsForDimension1=[-100,-60,-30,0,30,60,82.8,95]  Table=[-13.8,-10.1,-5.5,-0.4,7.4,13.85,15.7,15.7]  InternalRulePriority=Speed  RndMeth=Simplest  InputSameDT=on
  左轮上行 : Lookup_n-D  NumberOfTableDimensions=1  BreakpointsForDimension1=[-100,-60,-30,0,30,60,85,95]  Table=[-12.75,-9.7,-4.9,0.95,8.9,15.2,18,18.4]  InternalRulePriority=Speed  RndMeth=Simplest  InputSameDT=on
  左轮下行 : Lookup_n-D  NumberOfTableDimensions=1  BreakpointsForDimension1=[-100,-60,-30,0,30,60,84.6,95]  Table=[-12.5,-8.9,-4.55,0.85,9,15.4,18.35,18.35]  InternalRulePriority=Speed  RndMeth=Simplest  InputSameDT=on
  油门输入1 : ec311lib/RapidECU_U34/01BasicInput/AnalogInput  channel=52:I_AN05_5V  sampletime=-1
      settings: SourceProductName=ECUCoder for S32K311
  油门输入2 : ec311lib/RapidECU_U34/01BasicInput/AnalogInput  channel=54:I_AN07_5V  sampletime=-1
      settings: SourceProductName=ECUCoder for S32K311
  点火开关 : ec311lib/RapidECU_U34/01BasicInput/SwitchInput  channel=102:I_SW18_H/HALL9  sampletime=-1
      settings: SourceProductName=ECUCoder for S32K311
  计算最大驱动力 : Subsystem  Commented=on
  计算理想横摆角速度和质心侧偏角 : Subsystem
  计算理想转速 : Subsystem  Commented=on
  预充开关 : ec311lib/RapidECU_U34/01BasicInput/SwitchInput  channel=40:I_SW13_H/HALL8  sampletime=-1
      settings: SourceProductName=ECUCoder for S32K311
  驱动防滑使能 : Subsystem  Commented=on
  CAN0 0x111 BMS CAN发送 : Outport
  CAN2 0x185 右前 : Outport  Port=2
  CAN2 0x184 左前 : Outport  Port=3
  CAN2 0x189 右后 : Outport  Port=4
  CAN2 0x188 左后 : Outport  Port=5
  CAN0 0x190 测试量 : Outport  Port=6
  CAN0 0x191 测试量 : Outport  Port=7
  CAN0 0x192 测试量 : Outport  Port=8
  CAN0 0x194 测试量 : Outport  Port=9
  CAN0 CAN1 0x556 各种量 : Outport  Port=10
  CAN0 CAN1 0x557 温度和油压 : Outport  Port=11
  CAN0 CAN1 0x558 AMK电机速度 : Outport  Port=12
  CAN0 CAN1 0x559 车辆信息 : Outport  Port=13
  CAN0 CAN1 0x55B 加速度信息 : Outport  Port=14
  CAN0 0x195 测试量 : Outport  Port=15
  CAN0 0x193 测试量 : Outport  Port=16
  CAN0 0x55C 电机电流信息 : Outport  Port=17
  CAN0 0x55E vSOC : Outport  Port=18
  tag scope: K3105_Alive=global
  wires:
  MeaModule49/1 -> [SC_TestPoint3]
  [Roll_Angle] -> MATLAB Function10/3(Roll_Angle)
  [AMKSpeed_RR] -> Max3/4
  [TempIGBT4] -> Max/4
  [Unit_Min_Voltage] -> Gain4/1
  [Max_Power] -> 功率限制/3("Power ")
  Bus Selector11/3 -> Saturation21/1  "<TempInverter>"
  CAN0to2Receive/4 -> Subsystem3/3(CAN Msg)
  Product/1 -> MeaModule23/1
  Subtract8/1 -> [MotorAlive]
  MeaModule12/1 -> [acc1]
  计算理想横摆角速度和质心侧偏角/2(side_slip_angle_d_rad) -> [Side_Slip_Angle_d]
  Constant4/1 -> Add2/2
  [AMKSpeed_FR] -> Max3/2
  Bus Selector11/2 -> Saturation20/1  "<TempIGBT>"
  [T_max] -> Gain18/1
  NOT/1 -> Data Type Conversion8/1
  Bus Selector9/4 -> Saturation16/1  "<TempMotor>"
  Saturation11/1 -> [TempIGBT1]
  Constant36/1 -> Divide5/1, Divide7/2
  MATLAB Function11/1(Velocity) -> Saturation38/1
  CAN0to2Receive10/4 -> Subsystem10/3(CAN Msg)
  Constant/1 -> Data Type Conversion5/1
  [acc2] -> MATLAB Function7/2(acc2)
  [MaxTempMotor] -> Saturation31/1
  [Torque_Algorithm] -> Switch/1
  [Yaw_Rate_filter] -> Gain46/1
  CAN0to2Receive5/4 -> Subsystem5/3(CAN Msg)
  [precharge_input] -> MATLAB Function6/3(start_input)
  [East_Speed_filter] -> MATLAB Function11/1(East_Speed)
  Saturation3/1 -> Saturation36/1
  If Action Subsystem21/1(standby) -> Merge6/3
  Gain35/1 -> 计算理想转速/3(steer_angle)
  SwitchInput9/1 -> MeaModule50/1
  [Yaw_Rate_d] -> Gain47/1
  [Side_Slip_Angle_d] -> Gain44/1
  [AMK_bError_284] -> NOT1/1
  Bus Selector10/4 -> Saturation19/1  "<TempMotor>"
  [velocity] -> Gain17/1
  From38/1 -> Gain16/1
  [Side_Slip_Angle] -> Gain43/1
  [velocity] -> Gain45/1
  Product8/1 -> MeaModule70/1
  MeaModule45/1 -> Terminator17/1
  Data Type Conversion14/1 -> MeaModule20/1
  [acc_out] -> Product/2
  From33/1 -> Abs9/1
  Gain15/1 -> MATLAB Function2/2(Pitch_Angle)
  [brake] -> MATLAB Function5/6(break_state)
  From177/1 -> 计算理想转速/1(velocity)
  Tapped Delay8/1 -> Sum of Elements8/1
  If Action Subsystem20/1(ready_to_go) -> Merge6/2
  CAN0to2Receive7/3 -> Subsystem7/2(CAN ID)
  [TempInverter2] -> Max1/2
  MeaModule63/1 -> [Torque_FL_test]
  [TempInverter1] -> Max1/1
  Constant6/1 -> 功率限制1/3(DeratingRatio)
  MeaModule70/1 -> Saturation2/1
  MATLAB Function/1(avg) -> Gain19/1, [torque]
  Data Type Conversion10/1 -> MeaModule9/1
  Max3/1 -> Saturation29/1
  [AMKSpeed_RL] -> Max3/3
  Saturation27/1 -> MeaModule19/1
  CAN0to2Receive2/3 -> Subsystem2/2(CAN ID)
  MeaModule23/1 -> Saturation/1
  [TempMotor1] -> Max2/1
  From47/1 -> Gain14/1
  [TempIGBT2] -> Max/2
  [Torque_Normal] -> Switch/3
  Product2/1 -> MeaModule69/1
  CAN0to2Receive8/2 -> MeaModule15/1
  [acc] -> MATLAB Function/1(input_data)
  Gain3/1 -> AMKSpeed10/1
  If Action Subsystem9/1(Out1) -> Merge4/2
  If9/2 -> If Action Subsystem20/Action
  Gain9/1 -> Subtract8/3
  MeaModule42/1 -> [Heading_Angle]
  MeaModule/1 -> [acc]
  [AMKSpeed_RL] -> Abs2/1
  MeaModule33/1 -> Saturation1/1
  From90/1 -> Abs8/1
  Abs5/1 -> MATLAB Function5/5(yaw_rate_d)
  [iSOC] -> 1-D Lookup Table1/1
  MATLAB Function8/1(break_light) -> Data Type Conversion14/1
  MeaModule64/1 -> [Torque_RR_test]
  [Pitch_Angle] -> MATLAB Function10/2(Pitch_Angle)
  [acc_out] -> Product2/2
  Fcn1/1 -> MeaModule40/1
  left1/1 -> Saturation26/1
  Constant3/1 -> Subtract1/2
  Add2/1 -> Saturation34/1
  AnalogInput1/1 -> Saturation10/1
  Saturation39/1 -> MATLAB Function5/1(Torque_req)
  CAN0to2Receive/3 -> Subsystem3/2(CAN ID)
  [ControlMode] -> Bus Selector18/1
  From171/1 -> SMC_ASR/5(wheel_speed_d)
  Gain21/1 -> [T_max]
  Subtract1/1 -> mV_to %2/1
  [TargetVelocity] -> If Action Subsystem15/1(target_velocity)
  MeaModule50/1 -> [SC_TestPoint4]
  [Side_Slip_Angle_d] -> SMC/4(side_slip_angle_d)
  [Wheel_Steer_Angle] -> MATLAB Function5/3(steer_angle)
  If3/1 -> If Action Subsystem7/Action
  Saturation38/1 -> MeaModule55/1
  Subsystem10/1(BMS_data) -> Bus Selector13/1
  [T_max_d] -> MATLAB Function5/7(T_max)
  [AMKSpeed_RR] -> Abs3/1
  From34/1 -> 计算最大驱动力/1(torque)
  Bus Selector10/3 -> Saturation18/1  "<TempInverter>"
  [TempInverter4] -> Max1/4
  From170/1 -> SMC_ASR/2(yaw_rate_d)
  CAN0to2Receive10/3 -> Subsystem10/2(CAN ID)
  [TempIGBT1] -> Max/1
  [Torque] -> Demux1/1
  Divide7/1 -> Add3/1
  SMC_ASR/1(Turque_ASR) -> Goto46/1
  油门输入1/1 -> [acc1_input], Saturation3/1
  [TempIGBT3] -> Max/3
  [TempMotor4] -> Max2/4
  Bus Selector4/3 -> [AMKSpeed_FL]  "<AMK_Speed>"
  From174/1 -> SMC_ASR/4(wheel_speed), 计算最大驱动力/2(wheel_speed)
  [TempMotor3] -> Max2/3
  Saturation22/1 -> [TempMotor4]
  Saturation13/1 -> [TempMotor1]
  Bus Selector4/4 -> [AMK_bError_283]  "<bError>"
  Difference/1 -> MATLAB Function3/1(delta_angle)
  MeaModule29/1 -> PowerDriverSwitch(HS)/1
  CAN0to2Receive6/3 -> Subsystem6/2(CAN ID)
  Saturation35/1 -> MeaModule13/1
  Add1/1 -> Gain23/1
  [Yaw_Angle_filter] -> MATLAB Function4/2(Yaw_Angle)
  [Torque_RR] -> Product7/1
  Saturation29/1 -> [wheel_speed_max]
  Saturation33/1 -> MeaModule11/1
  [runflag] -> MATLAB Function6/1(runflag)
  MeaModule7/1 -> Subtract1/1
  CAN0to2Receive8/3 -> Subsystem11/2(CAN ID)
  Saturation31/1 -> 功率限制/1(MaxTempMotor)
  Subsystem7/1(28A_data) -> Bus Selector11/1
  Saturation30/1 -> [wheel_speed]
  [MaxTempMotor] -> 功率限制1/1(MaxTempMotor)
  MeaModule8/1 -> [precharge_input]
  From183/1 -> 驱动防滑使能/4(Torque)
  驱动防滑使能/2(ASR_Status) -> Goto118/1
  From184/1 -> 驱动防滑使能/1(Torque_ASR)
  Bus Selector8/2 -> Saturation11/1  "<TempIGBT>"
  [wheel_speed] -> 功率限制1/2(wheel_speed)
  Gain18/1 -> If Action Subsystem15/3(T_max)
  Mux3/1 -> Gain25/1
  [velocity] -> 计算理想横摆角速度和质心侧偏角/2(velocity_m/s)
  计算理想转速/1(wheel_speed_d) -> Goto45/1
  Gain19/1 -> [Torque_req]
  Bus Selector13/2 -> [BattTemp]  "<CellTemp>"
  Merge8/1 -> [DeratingRatio2]
  From41/1 -> 计算理想转速/2(Yaw_Rate), SMC_ASR/1(yaw_rate)
  MeaModule11/1 -> [acc2]
  [ControlMode] -> Bus Selector24/1
  CAN0to2Receive4/1 -> Subsystem12/Trigger
  MATLAB Function2/3(Acc_Z) -> MeaModule45/1
  CAN0to2Receive6/4 -> Subsystem6/3(CAN Msg)
  Abs9/1 -> Gain11/1
  [Mz] -> MATLAB Function5/2(Mz)
  [Torque_req] -> Saturation39/1
  [Yaw_Rate_d] -> Abs5/1
  MeaModule5/1 -> [start_input]
  [acc1] -> MATLAB Function7/1(acc1)
  [Heading_Angle] -> MATLAB Function4/1(Heading_Angle)
  If3/2 -> If Action Subsystem9/Action
  Gain36/1 -> 计算理想横摆角速度和质心侧偏角/1(steer_angle_rad)
  [Side_Slip_Angle] -> SMC/3(side_slip_angle)
  [Yaw_Rate_filter] -> Abs4/1
  [North_Speed_filter] -> MATLAB Function11/2(North_Speed)
  [Yaw_Rate_d] -> SMC/2(yaw_rate_d)
  [DeratingRatio2] -> MeaModule17/1
  [AMK_bError_287] -> NOT2/1
  MATLAB Function4/1(Side_Slip_Angle) -> MeaModule54/1
  [TempInverter3] -> Max1/3
  Bus Selector8/3 -> Saturation12/1  "<TempInverter>"
  NOT2/1 -> Data Type Conversion9/1
  [North_Speed_filter] -> MATLAB Function1/2(North_Speed)
  计算理想横摆角速度和质心侧偏角/1(yaw_rate_d_rad/s) -> [Yaw_Rate_d]
  NOT1/1 -> Data Type Conversion12/1
  MeaModule55/1 -> [velocity]
  From207/1 -> MATLAB Function2/5(Acc_Y_with_g)
  [Yaw_Angle] -> MATLAB Function10/1(Yaw_Angle)
  From29/1 -> Zero-Order Hold/1
  SwitchInput11/1 -> MeaModule46/1
  MeaModule44/1 -> Terminator16/1
  Gain37/1 -> [T_max_d]
  From42/1 -> MATLAB Function2/6(Acc_Z_with_g)
  MATLAB Function2/2(Acc_Y) -> MeaModule44/1
  MATLAB Function3/1(Yaw_Rate) -> MeaModule41/1
  mV_to %1/1 -> Saturation33/1
  StateChange2/3(beep) -> [beep]
  MeaModule41/1 -> Goto29/1
  Demux/1 -> Tapped Delay8/1
  Product7/1 -> MeaModule33/1
  [Yaw_Angle_filter] -> MATLAB Function1/3(Yaw_Angle)
  If Action Subsystem15/1(Torque_NegLimitRegene) -> [Torque_NegLimitRegene]
  [East_Speed_filter] -> MATLAB Function1/1(East_Speed)
  From28/1 -> Mux1/3
  If Action Subsystem15/2(Torque_Normal) -> [Torque_Normal]
  From27/1 -> Mux1/2
  CAN0to2Receive2/1 -> Subsystem2/Trigger
  [acc2_input] -> MATLAB Function9/2(acc2_input)
  Abs4/1 -> MATLAB Function5/4(yaw_rate)
  CAN0to2Receive3/2 -> Subsystem4/1(CAN_OK)
  [AMKSpeed_FR] -> Abs1/1
  Saturation15/1 -> [TempInverter2]
  Merge6/1 -> [ControlMode]
  StateChange2/2(readyLED_output) -> [readyLED_output]
  From158/1 -> Gain35/1
  If Action Subsystem22/1(Reset) -> Merge6/1
  [runflag] -> If3/1
  Data Type Conversion7/1 -> If9/1
  From15/1 -> Triggered Subsystem/Trigger
  Gain14/1 -> MATLAB Function2/1(Yaw_Angle)
  CAN0to2Receive3/3 -> Subsystem4/2(CAN ID)
  MeaModule69/1 -> Saturation5/1
  Saturation26/1 -> [vSOC]
  If9/1 -> If Action Subsystem22/Action
  MeaModule48/1 -> [SC_TestPoint2]
  Sum of Elements8/1 -> Gain39/1
  [ControlMode] -> Bus Selector20/1
  [SC_State] -> StateChange2/2(safe_input)
  Gain34/1 -> Gain38/1
  Gain38/1 -> [Torque_Algorithm], Demux/1
  Gain23/1 -> Add2/1
  MeaModule65/1 -> [Torque_RL_test]
  MeaModule1/1 -> Subtract3/1
  [Yaw_Rate_filter] -> SMC/1(yaw_rate)
  Abs8/1 -> Gain3/1
  From197/1 -> SMC_ASR/6(T_max)
  CAN0to2Receive/2 -> Subsystem3/1(CAN_OK)
  From172/1 -> 驱动防滑使能/3(wheel_speed_d)
  Saturation18/1 -> [TempInverter3]
  [wheel_speed_max] -> 功率限制/2(wheel_speed)
  MATLAB Function6/1(TargetVelocity) -> [TargetVelocity]
  Gain4/1 -> left1/1
  Saturation14/1 -> [TempIGBT2]
  油门输入2/1 -> [acc2_input], Saturation4/1
  [acc_flag] -> MATLAB Function6/2(acc_flag)
  功率限制1/1(T_max) -> Gain37/1
  If Action Subsystem7/1(Out1) -> Merge4/1
  Saturation20/1 -> [TempIGBT4]
  BRAKE_HIGH1/1 -> Subtract11/1
  CAN0to2Receive10/1 -> Subsystem10/Trigger
  Saturation34/1 -> MeaModule/1
  Add3/1 -> Saturation27/1
  NOT3/1 -> Data Type Conversion13/1
  Constant25/1 -> Add4/1, Add3/2
  Saturation10/1 -> Divide5/2
  From37/1 -> Gain15/1
  MeaModule6/1 -> [MaxTempIGBT]
  Subsystem12/1(285_data) -> Bus Selector8/1
  Saturation28/1 -> MeaModule27/1
  MeaModule40/1 -> Terminator10/1
  MATLAB Function1/1(Heading_Angle) -> MeaModule42/1
  Saturation32/1 -> MeaModule12/1
  [runflag] -> StateChange3/1(runflag)
  Gain10/1 -> Subtract8/4
  MeaModule54/1 -> Gain22/1
  Bus Selector9/1 -> [ErrorCode2]  "<ErrorCode>"
  Data Type Conversion9/1 -> Gain9/1
  [AMK_bError_288] -> NOT3/1
  CAN0to2Receive10/2 -> Subsystem10/1(CAN_OK)
  [AMK_bError_283] -> NOT/1
  CAN0to2Receive8/4 -> Subsystem11/3(CAN Msg)
  [Torque_Neg_RL] -> Saturation24/1
  Data Type Conversion13/1 -> Gain10/1
  MeaModule52/1 -> [MaxTempInverter]
  功率限制/1(T_max) -> Gain21/1
  From25/1 -> Mux1/1
  [readyLED_output] -> MeaModule29/1
  Saturation12/1 -> [TempInverter1]
  CAN0to2Receive5/3 -> Subsystem5/2(CAN ID)
  AnalogInput/1 -> Saturation9/1
  计算最大驱动力/1(Fx_max) -> SMC_ASR/3(Fx_max)
  Saturation17/1 -> [TempIGBT3]
  Max/1 -> MeaModule6/1
  If Action Subsystem5/1(DeratingRatio) -> Merge8/1
  Bus Selector9/3 -> Saturation15/1  "<TempInverter>"
  [TempMotor2] -> Max2/2
  MATLAB Function5/1(Torque) -> [Torque_Dis]
  Bus Selector10/1 -> [ErrorCode3]  "<ErrorCode>"
  Saturation9/1 -> Divide7/1
  Bus Selector11/1 -> [ErrorCode4]  "<ErrorCode>"
  CAN0to2Receive7/4 -> Subsystem7/3(CAN Msg)
  Bus Selector11/4 -> Saturation22/1  "<TempMotor>"
  Subsystem6/1(289_data) -> Bus Selector10/1
  Bus Selector9/2 -> Saturation14/1  "<TempIGBT>"
  CAN0to2Receive7/1 -> Subsystem7/Trigger
  [AMKSpeed_FL] -> Max3/1
  [Torque_Neg_FL] -> Saturation23/1
  Bus Selector10/2 -> Saturation17/1  "<TempIGBT>"
  CAN0to2Receive6/2 -> Subsystem6/1(CAN_OK)
  CAN0to2Receive6/1 -> Subsystem6/Trigger
  Divide5/1 -> Add4/2
  Subsystem5/1(286_data) -> Bus Selector9/1
  CAN0to2Receive5/1 -> Subsystem5/Trigger
  CAN0to2Receive4/4 -> Subsystem12/3(CAN Msg)
  AMKSpeed10/1 -> Bus Selector27/1
  CAN0to2Receive5/2 -> Subsystem5/1(CAN_OK)
  Bus Selector8/4 -> Saturation13/1  "<TempMotor>"
  [acc1_input] -> MATLAB Function9/1(acc1_input)
  Add4/1 -> Saturation28/1
  [Torque_FR] -> Product/1
  Bus Selector8/1 -> [ErrorCode1]  "<ErrorCode>"
  CAN0to2Receive4/2 -> Subsystem12/1(CAN_OK)
  CAN0to2Receive2/4 -> Subsystem2/3(CAN Msg)
  CAN0to2Receive3/1 -> Subsystem4/Trigger
  Bus Selector13/1 -> [BMS_State]  "<BMSState>"
  CAN0to2Receive4/3 -> Subsystem12/2(CAN ID)
  CAN0to2Receive2/2 -> Subsystem2/1(CAN_OK)
  [acc1] -> Add1/1
  [Wheel_Steer_Angle] -> Gain36/1
  CAN0to2Receive3/4 -> Subsystem4/3(CAN Msg)
  Gain11/1 -> AMKSpeed10/2
  MeaModule53/1 -> [MaxTempMotor]
  [start_input] -> StateChange3/2(start_input)
  Saturation21/1 -> [TempInverter4]
  CAN0to2Receive1/1 -> Subsystem1/Trigger
  Gain6/1 -> [Voltage]
  MeaModule47/1 -> [SC_TestPoint1]
  [brake] -> StateChange2/5(break_output)
  MeaModule46/1 -> [SC_State]
  mV_to %2/1 -> Saturation32/1
  Gain8/1 -> Subtract8/2
  Zero-Order Hold/1 -> Difference/1
  MeaModule13/1 -> [brake]
  点火开关/1 -> MeaModule5/1
  MeaModule26/1 -> [reset_input]
  Gain22/1 -> [Side_Slip_Angle]
  SwitchInput6/1 -> MeaModule47/1
  Saturation19/1 -> [TempMotor3]
  PowerVoltageMonitor/1 -> Data Type Conversion/1
  MeaModule43/1 -> Terminator11/1
  [start_input] -> StateChange2/4(start_input)
  Saturation16/1 -> [TempMotor2]
  SwitchInput7/1 -> MeaModule48/1
  Gain16/1 -> MATLAB Function2/3(Roll_Angle)
  [brake] -> MATLAB Function8/1(break_input)
  Max1/1 -> MeaModule52/1
  From39/1 -> MATLAB Function2/4(Acc_X_with_g)
  From182/1 -> 驱动防滑使能/2(wheel_speed)
  If Action Subsystem16/1(DeratingRatio) -> Merge8/2
  Data Type Conversion/1 -> Gain6/1
  [torque] -> Product1/2
  StateChange2/1(runflag) -> MeaModule2/1
  Data Type Conversion8/1 -> Gain7/1
  Subtract11/1 -> mV_to %/1
  Data Type Conversion6/1 -> PowerDriverSwitch(HS)2/1
  AMK复位开关/1 -> MeaModule26/1
  [precharge_input] -> StateChange2/3(precharge_input)
  Subsystem3/1(283_data) -> Bus Selector4/1
  Mux1/1 -> Fcn1/1
  MeaModule17/1 -> [DeratingRatio]
  [runflag] -> If9/2
  MeaModule62/1 -> [Torque_FR_test]
  [reset_input] -> StateChange3/3(reset_input)
  预充开关/1 -> MeaModule8/1
  [ControlMode] -> Bus Selector22/1
  [Torque_FL] -> Product2/1
  [Torque_RL] -> Product8/1
  SwitchInput8/1 -> MeaModule49/1
  Product1/1 -> If Action Subsystem15/2(torque)
  [Torque_Neg_RR] -> Saturation25/1
  [AMKSpeed_FL] -> Abs/1
  StateChange3/1(one_motor) -> [one_motor]
  [iSOC] -> If Action Subsystem5/1(In1)
  SwitchInput10/1 -> MeaModule51/1
  Max2/1 -> MeaModule53/1
  CAN0to2Receive/1 -> Subsystem3/Trigger
  Gain25/1 -> Saturation30/1
  MeaModule32/1 -> Saturation6/1
  1-D Lookup Table1/1 -> Saturation40/1
  [beep] -> Data Type Conversion6/1
  CAN0to2Receive7/2 -> Subsystem7/1(CAN_OK)
  [reset_input] -> Data Type Conversion7/1
  [iSOC] -> If7/1
  [Torque_req] -> Gain48/1
  Constant5/1 -> Product1/1
  Data Type Conversion12/1 -> Gain8/1
  [Torque_Neg_FR] -> Data Type Conversion2/1
  MeaModule27/1 -> [BreakPressure_R]
  CAN0to2Receive1/2 -> Subsystem1/1(CAN_OK)
  If7/2 -> If Action Subsystem16/Action
  If7/1 -> If Action Subsystem5/Action
  MeaModule20/1 -> PowerDriverSwitch(HS)1/1
  MeaModule19/1 -> [BreakPressure_F]
  [acc_flag] -> StateChange2/1(acc_flag)
  MeaModule2/1 -> [runflag]
  MeaModule51/1 -> [SC_TestPoint5]
  Data Type Conversion5/1 -> CAN5WakeUp/1
  Gain7/1 -> Subtract8/1
  MATLAB Function2/1(Acc_X) -> MeaModule43/1
  Merge4/1 -> CAN0 0x111 BMS CAN发送/1
  Bus Selector27/1 -> ?  "<Data>"
  [East_Speed] -> Subsystem/1(In1)
  [North_Speed] -> Subsystem/2(In2)
  [Yaw_Angle] -> Subsystem/3(In3)
  [Pitch_Angle] -> Subsystem/4(In4)
  [Roll_Angle] -> Subsystem/5(In5)
  [Yaw_Rate] -> Subsystem/6(In6)
  [INS_IMUAccrnX] -> Subsystem/7(In7)
  [INS_IMUAccrnY] -> Subsystem/8(In8)
  Subsystem/1(Out1) -> [East_Speed_filter]
  Subsystem/2(Out2) -> [North_Speed_filter]
  Subsystem/3(Out3) -> [Yaw_Angle_filter]
  Subsystem/4(Out4) -> [Pitch_Angle_filter]
  Subsystem/5(Out5) -> [Roll_Angle_filter]
  Subsystem/6(Out6) -> [Yaw_Rate_filter]
  Subsystem/7(Out7) -> [INS_IMUAccrnX_filter]
  Subsystem/8(Out8) -> [INS_IMUAccrnY_filter]
  [K3105G_flag] -> Subsystem/9(In9)
  MATLAB Function7/1(acc_flag) -> Data Type Conversion10/1
  MATLAB Function10/1(K3105G_flag) -> [K3105G_flag]
  Saturation6/1 -> Bus Creator1/6  "NegTorque"
  Saturation/1 -> Bus Creator1/7  "PosTorque"
  MeaModule31/1 -> Data Type Conversion11/1
  Bus Selector18/4 -> Bus Creator1/4  "<InverterOn>"
  Bus Selector18/3 -> Bus Creator1/3  "<ErrorReset>"
  Bus Selector18/2 -> Bus Creator1/2  "<Enable>"
  Bus Selector18/1 -> Bus Creator1/1  "<DcOn>"
  Bus Creator1/1 -> CAN2 0x185 右前/1
  Bus Creator2/1 -> CAN2 0x189 右后/1
  Saturation1/1 -> Bus Creator2/7  "PosTorque"
  Saturation25/1 -> Bus Creator2/6  "NegTorque"
  [TargetVelocity] -> Bus Creator2/5  "TargetVelocity"
  Bus Selector22/4 -> Bus Creator2/4  "<InverterOn>"
  Bus Selector22/3 -> Bus Creator2/3  "<ErrorReset>"
  Bus Selector22/2 -> Bus Creator2/2  "<Enable>"
  Bus Selector22/1 -> Bus Creator2/1  "<DcOn>"
  Saturation23/1 -> Bus Creator3/6  "NegTorque"
  Saturation5/1 -> Bus Creator3/7  "PosTorque"
  Bus Creator3/1 -> CAN2 0x184 左前/1
  [TargetVelocity] -> Bus Creator3/5  "TargetVelocity"
  Bus Selector20/4 -> Bus Creator3/4  "<InverterOn>"
  Bus Selector20/3 -> Bus Creator3/3  "<ErrorReset>"
  Bus Selector20/2 -> Bus Creator3/2  "<Enable>"
  Bus Selector20/1 -> Bus Creator3/1  "<DcOn>"
  Saturation24/1 -> Bus Creator4/6  "NegTorque"
  [TargetVelocity] -> Bus Creator4/5  "TargetVelocity"
  Bus Selector24/4 -> Bus Creator4/4  "<InverterOn>"
  Bus Selector24/3 -> Bus Creator4/3  "<ErrorReset>"
  Bus Selector24/2 -> Bus Creator4/2  "<Enable>"
  Bus Selector24/1 -> Bus Creator4/1  "<DcOn>"
  Saturation2/1 -> Bus Creator4/7  "PosTorque"
  Bus Creator4/1 -> CAN2 0x188 左后/1
  Bus Creator/1 -> CAN0 0x190 测试量/1
  [Torque_FL_test] -> Bus Creator/1  "TorqueFL"
  [Torque_FR_test] -> Bus Creator/2  "TorqueFR"
  [Torque_RL_test] -> Bus Creator/3  "TorqueRL"
  [Torque_RR_test] -> Bus Creator/4  "TorqueRR"
  [K3105G_flag] -> Bus Creator5/2  "K3105G_flag"
  [Mz] -> Bus Creator5/3  "Mz"
  Gain43/1 -> Bus Creator5/4  "SideSlipAngle"
  Gain44/1 -> Bus Creator5/5  "SideSlipAngle_d"
  Gain45/1 -> Bus Creator5/6  "velocity"
  Gain46/1 -> Bus Creator5/7  "YawRate"
  Gain47/1 -> Bus Creator5/8  "YawRate_d"
  Bus Creator5/1 -> CAN0 0x191 测试量/1
  [wheel_speed] -> CAN0 0x192 测试量/1
  Gain48/1 -> Bus Creator6/2  "Throttle"
  [brake] -> Bus Creator6/3  "Break"
  [Wheel_Steer_Angle] -> Bus Creator6/1  "SteeringAngle"
  Bus Creator6/1 -> CAN0 0x194 测试量/1
  Abs/1 -> Bus Creator7/1  "AMKSpeedFL"
  Abs1/1 -> Bus Creator7/2  "AMKSpeedFR"
  Abs2/1 -> Bus Creator7/3  "AMKSpeedRL"
  Abs3/1 -> Bus Creator7/4  "AMKSpeedRR"
  Bus Creator7/1 -> CAN0 CAN1 0x558 AMK电机速度/1
  [BMS_State] -> Bus Creator8/1  "BMSState"
  [ErrorCode1] -> Bus Creator8/2  "ErrorCode1"
  [ErrorCode2] -> Bus Creator8/3  "ErrorCode2"
  [ErrorCode3] -> Bus Creator8/4  "ErrorCode3"
  [ErrorCode4] -> Bus Creator8/5  "ErrorCode4"
  [SC_State] -> Bus Creator8/6  "SCState"
  [SC_TestPoint1] -> Bus Creator8/7  "SCTestPoint1"
  [SC_TestPoint2] -> Bus Creator8/8  "SCTestPoint2"
  [SC_TestPoint3] -> Bus Creator8/9  "SCTestPoint3"
  [SC_TestPoint4] -> Bus Creator8/10  "SCTestPoint4"
  [SC_TestPoint5] -> Bus Creator8/11  "SCTestPoint5"
  [Voltage] -> Bus Creator8/12  "Voltage"
  Bus Creator8/1 -> CAN0 CAN1 0x556 各种量/1
  [brake] -> Bus Creator9/1  "Break"
  [MotorAlive] -> Bus Creator9/2  "MotorAlive"
  [CarPower] -> Bus Creator9/3  "Power"
  [runflag] -> Bus Creator9/4  "runflag"
  [iSOC] -> Bus Creator9/5  "SOC"
  Gain17/1 -> Bus Creator9/6  "velocity"
  [Steer] -> Bus Creator9/7  "SteerAngle"
  [acc] -> Bus Creator9/8  "Throttle"
  [precharge_input] -> Bus Creator9/9  "PrechargeInput"
  [start_input] -> Bus Creator9/10  "StartInput"
  [reset_input] -> Bus Creator9/11  "ResetInput"
  Bus Creator9/1 -> CAN0 CAN1 0x559 车辆信息/1
  Bus Creator10/1 -> CAN0 CAN1 0x557 温度和油压/1
  [MaxTempIGBT] -> Bus Creator10/1  "IGBTTemp"
  [MaxTempInverter] -> Bus Creator10/2  "InverterTemp"
  [MaxTempMotor] -> Bus Creator10/3  "MotorTemp"
  [BattTemp] -> Bus Creator10/4  "BattTemp"
  [BreakPressure_F] -> Bus Creator10/5  "BreakPressureF"
  [BreakPressure_R] -> Bus Creator10/6  "BreakPressureR"
  [INS_IMUAccrnX] -> Bus Creator12/1  "AccX"
  [INS_IMUAccrnY] -> Bus Creator12/2  "AccY"
  Bus Creator12/1 -> CAN0 CAN1 0x55B 加速度信息/1
  [reset_input] -> StateChange4/3(reset_input)
  [precharge_input] -> StateChange4/2(precharge_input)
  [runflag] -> StateChange4/1(runflag)
  Constant10/1 -> Bus Creator10/7  "Algorithm_Enable"
  Logical Operator14/1 -> MATLAB Function12/1(K3105G_flag)
  Constant11/1 -> MATLAB Function12/2(Algorithm_Enable)
  [runflag] -> MATLAB Function12/3(Runflag)
  MATLAB Function12/1(flag) -> Switch/2
  [Steer] -> If Action Subsystem15/4(steer)
  Sum of Elements1/1 -> Gain27/1
  Sum of Elements/1 -> Gain26/1
  Tapped Delay1/1 -> Sum of Elements1/1
  Tapped Delay/1 -> Sum of Elements/1
  [AMKSpeed_FR] -> Tapped Delay/1
  [AMKSpeed_FL] -> Tapped Delay1/1
  Tapped Delay2/1 -> Sum of Elements2/1
  Sum of Elements2/1 -> Gain28/1
  [AMKSpeed_RR] -> Tapped Delay2/1
  Tapped Delay3/1 -> Sum of Elements3/1
  Sum of Elements3/1 -> Gain29/1
  [AMKSpeed_RL] -> Tapped Delay3/1
  [Torque_req] -> Gain30/1
  MATLAB Function13/1(factor_F) -> MATLAB Function5/8(factor_F)
  驱动防滑使能/1(Torque_Out) -> Terminator2/1
  Gain30/1 -> MATLAB Function14/1(Throttle), MATLAB Function13/1(Throttle)
  MATLAB Function14/1(factor_R) -> MATLAB Function5/9(factor_R)
  StateChange4/1(Algorithm_Enable) -> MeaModule14/1
  Constant8/1 -> Bus Creator5/1  "Algorithm_Enable"
  Sum of Elements4/1 -> Gain31/1
  Tapped Delay4/1 -> Sum of Elements4/1
  [Steer] -> Tapped Delay4/1
  [Yaw_Rate_filter] -> 计算理想横摆角速度和质心侧偏角/3(Yaw_Rate)
  [Side_Slip_Angle] -> 计算理想横摆角速度和质心侧偏角/4(Side_Slip_Angle)
  [K3105G_flag] -> 计算理想横摆角速度和质心侧偏角/5(K3105G_flag)
  Gain31/1 -> 右轮上行/1, 右轮下行/1, 左轮上行/1, 左轮下行/1
  左轮上行/1 -> Add/1
  左轮下行/1 -> Add/2
  右轮上行/1 -> Add/3
  右轮下行/1 -> Add/4
  Add/1 -> Gain32/1
  Gain32/1 -> [Wheel_Steer_Angle]
  [Yaw_Angle_filter] -> Bus Creator13/1  "Yaw_Angle"
  [Pitch_Angle_filter] -> Bus Creator13/2  "Pitch_Angle"
  [Roll_Angle_filter] -> Bus Creator13/3  "Roll_Angle"
  Bus Creator13/1 -> CAN0 0x195 测试量/1
  Bus Selector12/1 -> MeaModule22/1  "<IVT_MsgCount>"
  CAN0to2Receive9/1 -> Subsystem8/Trigger
  CAN0to2Receive9/4 -> Subsystem8/3(CAN Msg)
  CAN0to2Receive9/3 -> Subsystem8/2(CAN ID)
  CAN0to2Receive9/2 -> Subsystem8/1(CAN_OK)
  Bus Selector12/2 -> MeaModule21/1  "<IVT_Msg_Result_W>"
  MeaModule21/1 -> Gain2/1
  Subsystem8/1(IVT_data) -> Bus Selector12/1
  Gain2/1 -> [CarPower]
  MeaModule22/1 -> Terminator4/1
  Constant7/1 -> [acc_flag], [acc_out]
  [one_motor] -> Bus Creator10/8  "One_Motor"
  [Yaw_Rate_filter] -> Abs6/1
  [Yaw_Rate_d] -> Abs7/1
  Abs6/1 -> Subtract2/1
  Abs7/1 -> Subtract2/2
  Subtract2/1 -> Gain42/1
  Bus Creator14/1 -> CAN0 0x193 测试量/1
  From232/1 -> Mux2/4
  From235/1 -> Mux2/3
  From234/1 -> Mux2/2
  From233/1 -> Mux2/1
  Mux2/1 -> Abs10/1
  Abs10/1 -> Goto/1
  Demux2/1 -> Goto23/1
  Demux2/2 -> Goto120/1
  Demux2/3 -> Goto121/1
  Demux2/4 -> Goto122/1
  Data Type Conversion11/1 -> Bus Creator1/5  "TargetVelocity"
  From255/1 -> Subsystem17/7(Mz_r)
  Subsystem17/1(Tx) -> Goto125/1
  From247/1 -> Subsystem17/6(steer_angle)
  [INS_IMUAccrnY_filter] -> Subsystem15/2(acc_y)
  From26/1 -> Subsystem17/2(yaw_rate)
  From245/1 -> Subsystem17/1(Fz)
  From252/1 -> Subsystem17/5(T_max)
  From241/1 -> SMC_yaw_rate/4(steer_angle)
  From239/1 -> Subsystem17/3(yaw_rate_d)
  [INS_IMUAccrnX_filter] -> Subsystem15/1(acc_x)
  Subsystem15/1(Fz) -> [Fz]
  From248/1 -> Subsystem17/4(Torque_req)
  From243/1 -> SMC_yaw_rate/3(side_slip_angle)
  From242/1 -> SMC_yaw_rate/5(velocity)
  From246/1 -> Subsystem17/8(break_state)
  From240/1 -> SMC_yaw_rate/2(yaw_rate_d)
  From244/1 -> SMC_yaw_rate/1(yaw_rate)
  Demux3/1 -> Bus Creator14/1  "Fz_FL"
  Demux3/2 -> Bus Creator14/2  "Fz_FR"
  Demux3/3 -> Bus Creator14/3  "Fz_RL"
  Demux3/4 -> Bus Creator14/4  "Fz_RR"
  [Fz] -> Demux3/1
  Gain39/1 -> MeaModule63/1
  Gain27/1 -> Mux3/1
  Gain26/1 -> Mux3/2
  Gain28/1 -> Mux3/4
  Gain29/1 -> Mux3/3
  MeaModule16/1 -> Bus Creator6/4  "delta_YawRate"
  Demux/2 -> Tapped Delay5/1
  Gain33/1 -> MeaModule62/1
  Demux/3 -> Tapped Delay6/1
  Gain40/1 -> MeaModule65/1
  Demux/4 -> Tapped Delay7/1
  Gain41/1 -> MeaModule64/1
  SMC/1(ΔMz) -> MeaModule68/1
  MeaModule68/1 -> [Mz]
  [Torque_Dis] -> Gain34/1
  MeaModule25/1 -> Goto124/1
  SMC_yaw_rate/1(Mz_r) -> MeaModule25/1
  Demux1/2 -> [Torque_FR]
  Demux1/1 -> [Torque_FL]
  Demux1/4 -> [Torque_RR]
  Demux1/3 -> [Torque_RL]
  [TargetVelocity] -> MeaModule31/1
  [reset_input] -> StateChange5/1(reset_input)
  StateChange5/1(reset_state) -> [reset_state]
  [reset_state] -> MATLAB Function6/4(reset_state)
  [reset_state] -> If Action Subsystem15/5(reset_state)
  [runflag] -> StateChange5/2(run_flag)
  Gain42/1 -> MeaModule16/1
  Sum of Elements5/1 -> Gain33/1
  Tapped Delay5/1 -> Sum of Elements5/1
  Tapped Delay6/1 -> Sum of Elements6/1
  Sum of Elements6/1 -> Gain40/1
  Sum of Elements7/1 -> Gain41/1
  Tapped Delay7/1 -> Sum of Elements7/1
  [BMS_State] -> StateChange2/6(BMS_state)
  Saturation36/1 -> MeaModule7/1
  Saturation4/1 -> Saturation37/1
  Saturation37/1 -> MeaModule1/1
  Constant9/1 -> Subtract3/2
  Subtract3/1 -> mV_to %1/1
  刹车输入/1 -> Saturation41/1
  mV_to %/1 -> Saturation35/1
  Bus Selector1/2 -> Gain50/1  "<INS_IMUAccrnY>"
  [K3105_Alive] -> Logical Operator5/1
  Logical Operator12/1 -> Product16/2
  Gain50/1 -> Product4/1
  MeaModule74/1 -> [INS_IMUAccrnX]
  MeaModule83/1 -> [K3105_Alive]
  Product14/1 -> MeaModule79/1
  Product9/1 -> MeaModule71/1
  Gain49/1 -> Product3/1
  CAN0to2Receive13/1 -> Function-Call Subsystem/Trigger
  Product10/1 -> MeaModule72/1
  Logical Operator11/1 -> Product15/2
  MeaModule76/1 -> Terminator13/1
  M64CAN3to5Receive3/1 -> Subsystem18/Trigger
  [K3105_Alive] -> Logical Operator9/1
  Logical Operator7/1 -> Product11/2
  Product16/1 -> MeaModule75/1
  Logical Operator1/1 -> Product3/2
  Product15/1 -> MeaModule78/1
  Bus Selector1/3 -> Gain51/1  "<INS_IMUAccrnZ>"
  [K3105_Alive] -> Logical Operator12/1
  [K3105_Alive] -> Logical Operator11/1
  [K3105_Alive] -> Logical Operator2/1
  Product5/1 -> MeaModule61/1
  Logical Operator10/1 -> Product14/2
  Bus Selector1/7 -> MeaModule73/1  "<CAN_OK>"
  [K3105_Alive] -> Logical Operator8/1
  Subsystem19/1(IMU_data) -> Bus Selector1/1
  Logical Operator8/1 -> Product12/2
  Product6/1 -> MeaModule67/1
  M64CAN3to5Receive2/2 -> Subsystem19/1(CAN_OK)
  Logical Operator3/1 -> Product5/2
  Product3/1 -> MeaModule74/1
  Product4/1 -> MeaModule82/1
  [K3105_Alive] -> Logical Operator4/1
  [K3105_Alive] -> Logical Operator3/1
  Gain52/1 -> [Yaw_Rate]
  [K3105_Alive] -> Logical Operator6/1
  Logical Operator6/1 -> Product10/2
  CAN0to2Receive13/2 -> Function-Call Subsystem/1(CAN_OK)
  Bus Selector/1 -> MeaModule83/1  "<K3105_Alive>"
  CAN0to2Receive13/4 -> Function-Call Subsystem/3(CAN_MSG)
  MeaModule71/1 -> Terminator8/1
  Bus Selector1/1 -> Gain49/1  "<INS_IMUAccrnX>"
  M64CAN3to5Receive2/4 -> Subsystem19/3(CAN Msg)
  Logical Operator9/1 -> Product13/2
  MeaModule81/1 -> [Roll_Angle]
  M64CAN3to5Receive3/4 -> Subsystem18/3(CAN Msg)
  CAN0to2Receive13/3 -> Function-Call Subsystem/2("CAN_ID ")
  MeaModule82/1 -> [INS_IMUAccrnY]
  Bus Selector2/2 -> Product15/1  "<East_Speed>"
  [K3105_Alive] -> Logical Operator1/1
  MeaModule80/1 -> [Pitch_Angle]
  Function-Call Subsystem/1(Dashboard_Control) -> Bus Selector/1
  Bus Selector2/5 -> Product12/1  "<Pitch_Angle>"
  Bus Selector2/6 -> Product11/1  "<Roll_Angle>"
  Bus Selector2/4 -> Product13/1  "<Heading_Angle>"
  Product13/1 -> MeaModule77/1
  Bus Selector2/7 -> MeaModule76/1  "<CAN_OK>"
  MeaModule61/1 -> [INS_IMUAccrnZ]
  MeaModule72/1 -> Gain52/1
  M64CAN3to5Receive2/1 -> Subsystem19/Trigger
  M64CAN3to5Receive3/3 -> Subsystem18/2(CAN ID)
  Bus Selector1/5 -> Product9/1  "<INS_IMUAglRateY>"
  MeaModule79/1 -> [North_Speed]
  MeaModule78/1 -> [East_Speed]
  Gain51/1 -> Product5/1
  MeaModule67/1 -> Terminator7/1
  Bus Selector1/4 -> Product6/1  "<INS_IMUAglRateX>"
  MeaModule73/1 -> Terminator12/1
  Logical Operator4/1 -> Product6/2
  Logical Operator5/1 -> Product9/2
  Product12/1 -> MeaModule80/1
  MeaModule75/1 -> Terminator9/1
  Bus Selector1/6 -> Product10/1  "<INS_IMUAglRateZ>"
  M64CAN3to5Receive3/2 -> Subsystem18/1(CAN_OK)
  [K3105_Alive] -> Logical Operator7/1
  Bus Selector2/1 -> Product16/1  "<To_Ground_Speed>"
  M64CAN3to5Receive3/5 -> Subsystem18/4(DLC)
  Bus Selector2/3 -> Product14/1  "<North_Speed>"
  M64CAN3to5Receive2/5 -> Subsystem19/4(DLC)
  Logical Operator2/1 -> Product4/2
  Product11/1 -> MeaModule81/1
  MeaModule77/1 -> [Yaw_Angle]
  M64CAN3to5Receive2/3 -> Subsystem19/2(CAN ID)
  [K3105_Alive] -> Logical Operator10/1
  Subsystem18/1(GNSS_data) -> Bus Selector2/1
  MeaModule4/1 -> Subtract11/2
  If9/3 -> If Action Subsystem21/Action
  [acc2] -> Add1/2
  Logical Operator13/1 -> Logical Operator14/1
  [K3105_Alive] -> Logical Operator13/1
  [K3105G_flag] -> Logical Operator14/2
  Switch/1 -> [Torque]
  [BreakPressure_R] -> StateChange1/2(brake_pressure_r)
  [acc] -> StateChange1/1(acc)
  StateChange1/1(flag_regen) -> [flag_regen]
  [flag_regen] -> MATLAB Function6/5(flag_regen)
  [flag_regen] -> If Action Subsystem15/6(flag_regen)
  [iSOC] -> If Action Subsystem15/7(SOC)
  [BreakPressure_R] -> If Action Subsystem15/9(brake_pressure_r)
  Bus Selector4/1 -> [Id_283]  "<Id>"
  Bus Selector4/2 -> [Iq_283]  "<Iq>"
  Subsystem1/1(284_data) -> Bus Selector3/1
  CAN0to2Receive1/3 -> Subsystem1/2(CAN ID)
  CAN0to2Receive1/4 -> Subsystem1/3(CAN Msg)
  Bus Selector3/3 -> [AMKSpeed_FR]  "<AMK_Speed>"
  Bus Selector3/4 -> [AMK_bError_284]  "<bError>"
  Bus Selector3/1 -> [Id_284]  "<Id>"
  Bus Selector3/2 -> [Iq_284]  "<Iq>"
  Subsystem2/1(287_data) -> Bus Selector5/1
  Bus Selector5/3 -> [AMKSpeed_RL]  "<AMK_Speed>"
  Bus Selector5/4 -> [AMK_bError_287]  "<bError>"
  Bus Selector5/1 -> [Id_287]  "<Id>"
  Bus Selector5/2 -> [Iq_287]  "<Iq>"
  Subsystem4/1(288_data) -> Bus Selector6/1
  Bus Selector6/3 -> [AMKSpeed_RR]  "<AMK_Speed>"
  Bus Selector6/4 -> [AMK_bError_288]  "<bError>"
  Bus Selector6/1 -> [Id_288]  "<Id>"
  Bus Selector6/2 -> [Iq_288]  "<Iq>"
  [Iq_284] -> Bus Creator15/2  "Iq_284"
  [Id_284] -> Bus Creator15/1  "Id_284"
  Bus Creator15/1 -> CAN0 0x55C 电机电流信息/1
  [Torque_Neg_FR] -> Bus Creator15/4  "Torque_regen"
  [flag_regen] -> Bus Creator15/5  "flag_regen"
  [runflag] -> StateChange1/3(run_flag)
  [TargetVelocity] -> Bus Creator15/3  "Target_velocity"
  [wheel_speed_max] -> If Action Subsystem15/10(AMKSpeed)
  Bus Selector13/4 -> [Unit_Min_Voltage]  "<MinCellVolt>"
  Bus Selector13/5 -> [iSOC]  "<SOC>"
  Bus Selector13/3 -> [Unit_Max_Voltage]  "<MaxCellVolt>"
  [Unit_Max_Voltage] -> If Action Subsystem15/11(MaxCellVolt)
  Subsystem11/1(steer_angle_data) -> MeaModule66/1
  CAN0to2Receive8/1 -> Subsystem11/Trigger
  MeaModule9/1 -> Goto137/1
  MATLAB Function9/1(acc_out) -> Goto138/1
  Product17/1 -> MeaModule10/1
  MATLAB Function16/1(avg) -> MeaModule4/1
  Data Type Conversion1/1 -> MATLAB Function16/1(input_data)
  Saturation41/1 -> Data Type Conversion1/1
  [vSOC] -> Bus Creator11/1  "vSOC"
  Bus Creator11/1 -> CAN0 0x55E vSOC/1
  Saturation40/1 -> [Max_Power]
  [BreakPressure_F] -> If Action Subsystem15/8(brake_pressure_f)
  [Torque_NegLimitRegene] -> Demux4/1
  Demux4/1 -> [Torque_Neg_FL]
  Demux4/2 -> [Torque_Neg_FR]
  Demux4/3 -> [Torque_Neg_RL]
  Demux4/4 -> [Torque_Neg_RR]
  [acc_out] -> Product7/2
  [acc_out] -> Product8/2
  [one_motor] -> Product/3
  [one_motor] -> Product2/3
  Data Type Conversion2/1 -> MeaModule32/1
  MeaModule66/1 -> Add5/1
  Add5/1 -> Product17/1
  Constant2/1 -> Add5/2
  [Algorithm_Enable] -> Logical Operator15/1
  Logical Operator15/1 -> Product17/2
  MeaModule10/1 -> [Steer]
  MeaModule14/1 -> [Algorithm_Enable]
  MeaModule15/1 -> Subsystem11/1(CAN_OK)
